simulink model "PIDEstimator"  (Simulink 10.0)
settings: Solver=ode3  StartTime=0.0  StopTime=Tsim  FixedStep=deltat  RelTol=1e-3  EnableMultiTasking=on
values from neighbouring files (symbols this model uses):
  a0 = -1    [estimator_params_pid.m]
  a1 = 0    [estimator_params_pid.m]
  alpha3 = 4    [estimator_params_pid.m]
  delay = 0.01    [estimator_params_pi.m]    (also in estimator_params_pid.m)
  deltat = 0.001    [estimator_params_pi.m]    (also in estimator_params_pid.m)
  Gs = tf(2, [1 0 -1])    [estimator_params_pid.m]    (also in params.m = tf(88, [170 1]))
  K1 = 10    [estimator_params_pi.m]    (also in estimator_params_pid.m = 5)
  K2 = 30    [estimator_params_pi.m]    (also in estimator_params_pid.m = 2.121)
  K3 = 2    [estimator_params_pid.m]
  tauf = 0.1*taud    (= 0.04242)    [estimator_params_pid.m]
  Tsim = 20    [estimator_params_pi.m]    (also in estimator_params_pid.m)
  umax = 41.9*0.85    (= 35.615)    [estimator_params_pi.m]    (also in estimator_params_pid.m = 999)
  umin = -9    [estimator_params_pi.m]    (also in estimator_params_pid.m = -999)
settings Model: Creator=e50128  LastModifiedBy=adityaaaap
settings DataIOCC: LimitDataPoints=on  SignalLoggingSaveFormat=ModelDataLogs
settings OptimizationCC: ExpressionDepthLimit=2147483647
settings DebuggingCC: SolverPrmCheckMsg=warning  FcnCallInpInsideContextMsg=warning  StateNameClashWarn=warning
settings GRTTargetCC: GeneratePreprocessorConditionals=Disable all
settings ConfigComp: CovExternalEMLEnable=off

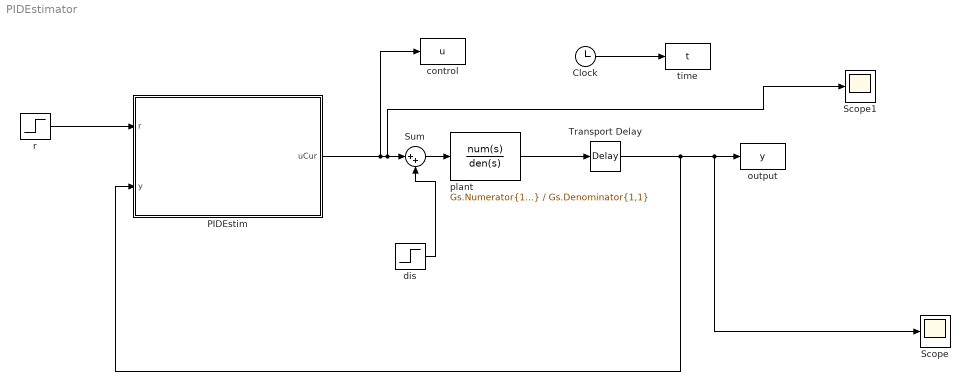
== system PIDEstimator ==
  Clock : Clock
  PIDEstim : MATLAB Function  TreatAsAtomicUnit=on
  Scope : Scope
  Scope1 : Scope
  Sum : Sum  Inputs=|++
  Transport Delay : TransportDelay  DelayTime=delay
  control : ToWorkspace  VariableName=u
      settings: MaxDataPoints=10000
  dis : Step  Time=Tsim/2  After=20  SampleTime=0
  output : ToWorkspace  VariableName=y
      settings: MaxDataPoints=10000
  plant : TransferFcn  Numerator=Gs.Numerator{1,1}  Denominator=Gs.Denominator{1,1}
  r : Step  Time=0  SampleTime=0
  time : ToWorkspace  VariableName=t
      settings: MaxDataPoints=10000
  wires:
  r/1 -> PIDEstim/1(r)
  Clock/1 -> time/1
  plant/1 -> Transport Delay/1
  PIDEstim/1(uCur) -> control/1, Scope1/1, Sum/1
  dis/1 -> Sum/2
  Sum/1 -> plant/1
  Transport Delay/1 -> Scope/1, output/1, PIDEstim/2(y)

== matlab function PIDEstim ==
  settings: updateMethod=DISCRETE  sampleTime=deltat
  data: uCur output double; r input double; y input double; K1 parameter double; K2 parameter double; K3 parameter double; tauf parameter double; alpha3 parameter double; a1 parameter double; a0 parameter double; deltat parameter double; umin parameter double; umax parameter double
function uCur = PIDEstFD(r,y,K1,K2,K3,tauf,alpha3,a1,a0,deltat,umin,umax)
persistent zhat
if isempty(zhat)
    zhat=0;
end
persistent ydfpast
if isempty(ydfpast)
    ydfpast=0;
end
persistent ypast
if isempty(ypast)
    ypast=0;
end


% ndmax=100; 
% persistent(udelay)
% if isempty(udelay)
%     udelay=zeros(1,ndmax);
% end   
%estimator based MATLAB function with anti-windup
ydf=tauf/(tauf+deltat)*ydfpast+1/(tauf+deltat)*(y-ypast); 
dhat=zhat+K3*ydf;   
uCur= -K1*(y-r)-K2*ydf-dhat;
if (uCur>umax) uCur=umax;end
if (uCur<umin) uCur=umin;end
zhat=zhat-deltat*alpha3*zhat+deltat*(K3*(a1-alpha3)*ydf+K3*a0*(y-r)-alpha3*uCur);
ypast=y;
ydfpast=ydf;
%udelay=[uCur udelay(1,1:ndmax-1)];
